simulink model "brightnessController_Harness1"  (R2020b)
settings: Solver=VariableStepAuto  StartTime=0.0  StopTime=10.0  RelTol=1e-3
settings Model: Creator=Balazs  LastModifiedBy=Balazs

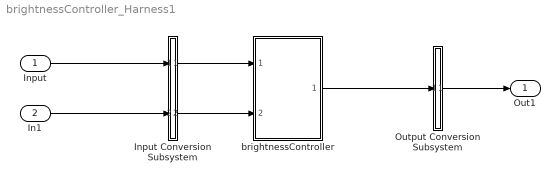
== system brightnessController_Harness1 ==
  Input : Inport  OutDataTypeStr=boolean  PortDimensions=[1]  SampleTime=[0, 1]
  In1 : Inport  Port=2  OutDataTypeStr=uint16  PortDimensions=[1]  SampleTime=[0, 1]
  Input Conversion Subsystem : Subsystem  Tag=__SLT_ICS__  Description=|
      | Signal spec.
      | and routing
      settings: AttributesFormatString=%<Description>
  Output Conversion Subsystem : Subsystem  Tag=__SLT_OCS__  Description=|
      | Signal spec.
      | and routing
      settings: AttributesFormatString=%<Description>
  brightnessController : ModelReference  ModelNameDialog=brightnessController  SimulationMode=Normal  ModelReferenceVersion=1.10
  Out1 : Outport
  wires:
  Input/1 -> Input Conversion Subsystem/1(Inport_1)
  In1/1 -> Input Conversion Subsystem/2(Inport_2)
  Output Conversion Subsystem/1(Outport_1) -> Out1/1
  Input Conversion Subsystem/1(Outport_1) -> brightnessController/1
  Input Conversion Subsystem/2(Outport_2) -> brightnessController/2
  brightnessController/1 -> Output Conversion Subsystem/1(Inport_1)

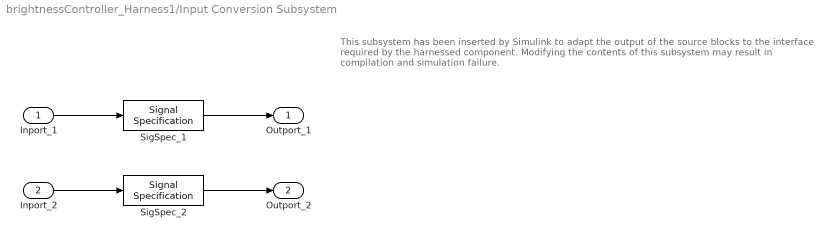
== system brightnessController_Harness1/Input Conversion Subsystem ==
  note: This subsystem has been inserted by Simulink to adapt the output of the source blocks to the interface required by the harnessed component.
      |  Modifying the contents of this subsystem may result in compilation and simulation failure.
  Inport_1 : Inport
  Inport_2 : Inport  Port=2
  SigSpec_1 : SignalSpecification  OutDataTypeStr=boolean  Dimensions=[1]  SampleTime=[0, 1]
  SigSpec_2 : SignalSpecification  OutDataTypeStr=uint16  Dimensions=[1]  SampleTime=[0, 1]
  Outport_1 : Outport
  Outport_2 : Outport  Port=2
  wires:
  SigSpec_1/1 -> Outport_1/1
  Inport_1/1 -> SigSpec_1/1
  SigSpec_2/1 -> Outport_2/1
  Inport_2/1 -> SigSpec_2/1

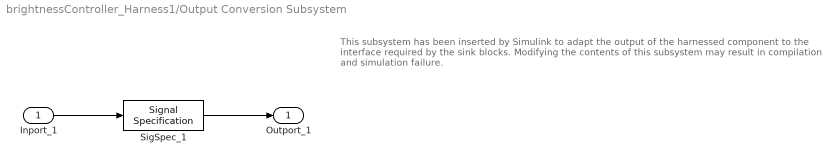
== system brightnessController_Harness1/Output Conversion Subsystem ==
  note: This subsystem has been inserted by Simulink to adapt the output of the harnessed component to the interface required by the sink blocks.
      |  Modifying the contents of this subsystem may result in compilation and simulation failure.
  Inport_1 : Inport
  SigSpec_1 : SignalSpecification  OutDataTypeStr=uint16  Dimensions=[1]
  Outport_1 : Outport
  wires:
  Inport_1/1 -> SigSpec_1/1
  SigSpec_1/1 -> Outport_1/1
